simulink model "DEA_strip_t2"  (R2018a)
settings: Solver=ode23t  StartTime=0.0  StopTime=50  EnableMultiTasking=on
InitFcn:
  | Parameter;
values from neighbouring files (symbols this model uses):
  param_f = 0.001    [plot_task2.m]
  param_g = 9.81    [plot_task2.m]
  param_k1 = 10800    [plot_task2.m]
  param_k2 = 43200    [plot_task2.m]
  param_m1 = 0.25    [plot_task2.m]
  param_m2 = 0.25    [plot_task2.m]
  param_N = 8    [plot_task2.m]
  param_y2 = -1.135*10^-4    (= -0.0001135)    [plot_task2.m]
  param_ys0 = 0.09    [plot_task2.m]
  params = struct    [Parameter_t2.m]
settings Model: Creator=Johannes  LastModifiedBy=Matthias
settings DataIOCC: LimitDataPoints=on  SaveFormat=Array  SignalLoggingSaveFormat=ModelDataLogs
settings OptimizationCC: LifeSpan=inf
settings DebuggingCC: UnderspecifiedInitializationDetection=Classic  MergeDetectMultiDrivingBlocksExec=none  SolverPrmCheckMsg=warning  MultiTaskDSMMsg=warning  MultiTaskCondExecSysMsg=none  SFUnexpectedBacktrackingDiag=warning  SFNoUnconditionalDefaultTransitionDiag=warning  SFExecutionAtInitializationDiag=none
settings HardwareCC: ProdBitPerPointer=32  ProdBitPerSizeT=32  ProdBitPerPtrDiffT=32  ProdLargestAtomicFloat=None  ProdIntDivRoundTo=Undefined  ProdEndianess=Unspecified  ProdWordSize=32  ProdHWDeviceType=32-bit Generic
settings ModelReferenceCC: PropagateSignalLabelsOutOfModel=off
settings CodeAppCC: StateflowObjectComments=on
settings GRTTargetCC: TargetLangStandard=C89/C90 (ANSI)  GeneratePreprocessorConditionals=Disable all
settings ConfigComp: CovMetricSettings=dw  CovHtmlReporting=on  CovSaveCumulativeToWorkspaceVar=on  CovSaveSingleToWorkspaceVar=on  CovExternalEMLEnable=off

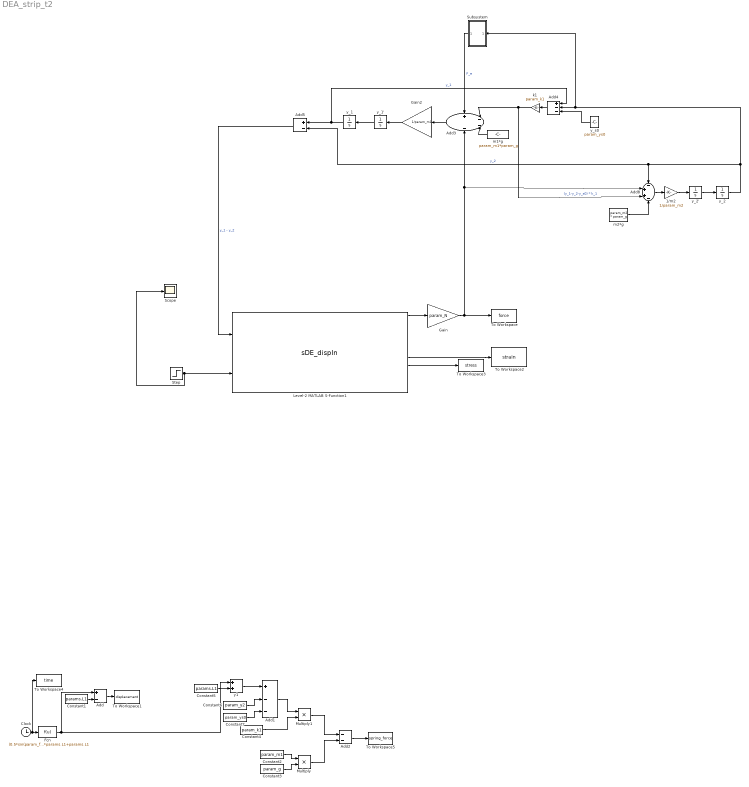
== system DEA_strip_t2 ==
  "1/m2 " : Gain  Gain=1/param_m2
  Add : Sum  Inputs=+-
  Add1 : Sum  Inputs=+--
  Add2 : Sum  Inputs=--
  Add3 : Sum  Inputs=+---
  Add4 : Sum  Inputs=+--
  Add5 : Sum  Inputs=+-
  Add8 : Sum  Inputs=-++-
  Clock : Clock
  Constant1 : Constant  Value=params.L1
  Constant2 : Constant  Value=param_m1
  Constant3 : Constant  Value=param_g
  Constant4 : Constant  Value=param_k1
  Constant5 : Constant  Value=params.L1
  Constant6 : Constant  Value=param_y2
  Constant7 : Constant  Value=param_ys0
  Fcn : Fcn  Expr=(0.5*sin(param_f*u)+0.5)*params.L1+params.L1
  Gain : Gain  Gain=param_N
  Gain2 : Gain  Gain=1/param_m1
  Level-2 MATLAB S-Function1 : M-S-Function  FunctionName=sDE_dispIn  Parameters=params, initConds
      mask Display:
      | color('black');
      | patch(4*[-1 1 1 -1],1.75*[-1 -1 1 1],[1 1 1]);
      | patch(2*[-1 1 1 -1],1.2*[-1 -1 1 1],[0 0 0]);
      | patch(1.95*[-1 1 1 -1],0.8*[-1 -1 1 1],[1 1 1]);
      | disp('DE Actuator');
      | 
      | color('blue');
      | port_label('input', 1, 'l_1 [m]','texmode','on');
      | port_label('input', 2, 'v [V]','texmode','on');
      | 
      | color('red');
      | port_label('output', 1, 'F_1 [N]','texmode','on');
      | port_label('output', 2, 'x_{v1} [-]','texmode','on');
      | port_label('output', 3, 'x_{v2} [-]','texmode','on');
      | port_label('output', 4, '\epsilon_2 [-]','texmode','on');
      | port_label('output', 5, 'q [C]','texmode','on');
      | port_label('output', 6, '\epsilon_1 [-]','texmode','on');
      | port_label('output', 7, '\sigma_1 [Pa]','texmode','on');
      | port_label('output', 8, 'i [A]','texmode','on');
      | port_label('output', 9, 'v_{DE} [V]','texmode','on');
      | port_label('output', 10, 'C [F]','texmode','on');
  Multiply : Product
  Multiply1 : Product
  Scope : Scope
  Step : Step  Time=5  After=2500  SampleTime=0
  Subsystem : Subsystem
  To Workspace : ToWorkspace  VariableName=force  SampleTime=-1
  To Workspace1 : ToWorkspace  VariableName=displacement  SampleTime=-1
  To Workspace2 : ToWorkspace  VariableName=strain  SampleTime=-1
  To Workspace3 : ToWorkspace  VariableName=stress  SampleTime=-1
  To Workspace4 : ToWorkspace  VariableName=time  SampleTime=-1
  To Workspace5 : ToWorkspace  VariableName=spring_force  SampleTime=-1
  k1 : Gain  Gain=param_k1
  m1*g : Constant  Value=param_m1*param_g
  m2*g : Constant  Value=param_m2 * param_g
  "y1 " : Sum
  y_1 : Integrator  InitialCondition=param_ys0
  y_1' : Integrator
  y_2 : Integrator  InitialCondition=0.03
  y_2' : Integrator
  y_s0 : Constant  Value=param_ys0
  wires:
  Clock/1 -> To Workspace4/1, Fcn/1
  Fcn/1 -> "y1 "/1, Add/1
  Level-2 MATLAB S-Function1/1 -> Gain/1
  Level-2 MATLAB S-Function1/6 -> To Workspace2/1
  Level-2 MATLAB S-Function1/7 -> To Workspace3/1
  Add/1 -> To Workspace1/1
  Constant1/1 -> Add/2
  Gain/1 -> Add8/2, Add3/4, To Workspace/1
  Constant2/1 -> Multiply/1
  Constant3/1 -> Multiply/2
  Constant5/1 -> "y1 "/2
  "y1 "/1 -> Add1/1
  Constant6/1 -> Add1/2
  Constant7/1 -> Add1/3
  Add1/1 -> Multiply1/1
  Constant4/1 -> Multiply1/2
  Add2/1 -> To Workspace5/1
  Multiply1/1 -> Add2/1
  Multiply/1 -> Add2/2
  m1*g/1 -> Add3/3
  y_s0/1 -> Add4/3
  Add3/1 -> Gain2/1
  Gain2/1 -> y_1'/1
  y_1'/1 -> y_1/1
  y_1/1 -> Add4/1, Add5/1  "y_1"
  y_2/1 -> Add8/1, Add5/2, Subsystem/1(y_2), Add4/2  "y_2"
  Add5/1 -> Level-2 MATLAB S-Function1/1  "y_1 - y_2"
  Add4/1 -> k1/1
  k1/1 -> Add8/3, Add3/2  "(y_1-y_2-y_s0) * k_1"
  Step/1 -> Scope/1, Level-2 MATLAB S-Function1/2
  m2*g/1 -> Add8/4
  y_2'/1 -> y_2/1
  Add8/1 -> "1/m2 "/1
  "1/m2 "/1 -> y_2'/1
  Subsystem/1(F_e) -> Add3/1  "F_e"

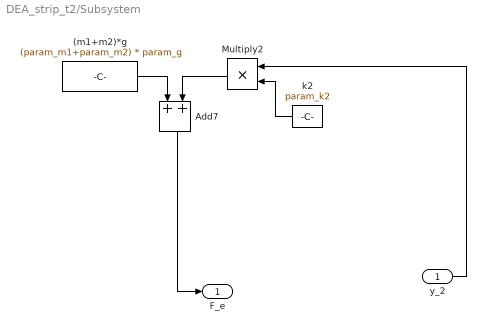
== system DEA_strip_t2/Subsystem ==
  y_2 : Inport
  (m1+m2)*g : Constant  Value=(param_m1+param_m2) * param_g
  Add7 : Sum
  Multiply2 : Product
  k2 : Constant  Value=param_k2
  F_e : Outport
  wires:
  (m1+m2)*g/1 -> Add7/1
  k2/1 -> Multiply2/2
  Add7/1 -> F_e/1
  Multiply2/1 -> Add7/2
  y_2/1 -> Multiply2/1
